simulink model "simulink_control"  (R2024a)
settings: Solver=ode5  StartTime=0.0  StopTime=inf  FixedStep=0.016  RelTol=1e-3
values from neighbouring files (symbols this model uses):
  hip = wb_robot_get_device('hip')    [inverted_pendulum_noncart.m]
  horizontal_motor = wb_robot_get_device('horizontal_motor')    [inverted_pendulum_noncart.m]
  horizontal_position_sensor = wb_robot_get_device('horizontal position sensor')    [inverted_pendulum_noncart.m]
  TIME_STEP = 16    [inverted_pendulum_noncart.m]
undefined symbols (not defined in the file or in its folder): a1, a2, a3, a4, accelerometer_sensor
libraries: slpidlib x2, eeGeneralControl x1, simulink_extras x1
settings Model: Creator=Harun  LastModifiedBy=Harun

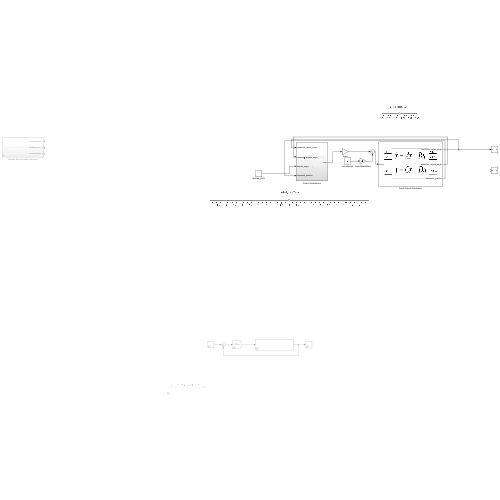
[thumbnail: Simulink's stored preview of the top-level diagram]
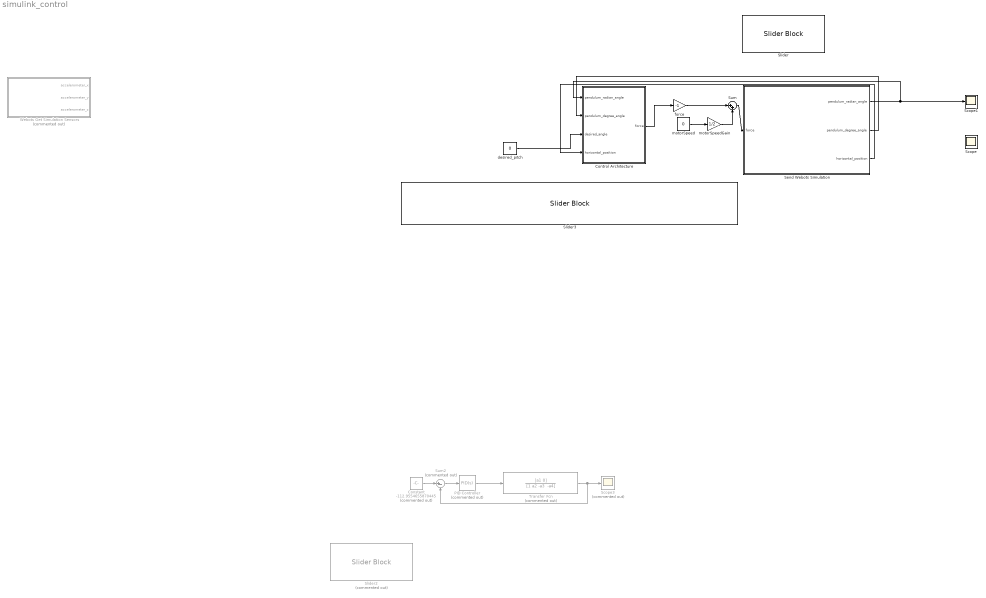
== system simulink_control ==
  Constant : Constant  Commented=on  Value=-112.9554655870445
  Control Architecture : Subsystem
  PID Controller : slpidlib/PID Controller  Commented=on  Controller=PID  Form=Parallel  TimeDomain=Continuous-time  UseExternalTs=off  SampleTime=-1  IntegratorMethod=Forward Euler  FilterMethod=Forward Euler  ControllerParametersSource=internal  P=117.155618821838  I=67.2944879318419  UseKiTs=off  D=44.7801205202101  UseExternalDerivativeSource=off  N=97.4887289682428  UseFilter=on  TunerSelectOption=Transfer Function Based (PID Tuner App)  InitialConditionSource=internal  InitialConditionForIntegrator=0  InitialConditionForFilter=0  DifferentiatorICPrevScaledInput=0  ExternalReset=none  TrackingMode=off  Kt=1  LimitOutput=off  SatLimitsSource=internal  UpperSaturationLimit=inf  LowerSaturationLimit=-inf  LinearizeAsGain=on  AntiWindupMode=none  Kb=1  LimitIntegrator=off  UpperIntegratorSaturationLimit=inf  LowerIntegratorSaturationLimit=-inf  POutMin=[]  POutMax=[]  IOutMin=[]  IOutMax=[]  DOutMin=[]  DOutMax=[]  NOutMin=[]  NOutMax=[]  SumOutMin=[]  SumOutMax=[]  SaturationOutMin=[]  SaturationOutMax=[]  PParamMin=[]  PParamMax=[]  IParamMin=[]  IParamMax=[]  DParamMin=[]  DParamMax=[]  NParamMin=[]  NParamMax=[]  KbParamMin=[]  KbParamMax=[]  KtParamMin=[]  KtParamMax=[]  KbOutMin=[]  KbOutMax=[]  KtOutMin=[]  KtOutMax=[]  IntegratorOutMin=[]  IntegratorOutMax=[]  FilterOutMin=[]  FilterOutMax=[]  SumI1OutMin=[]  SumI1OutMax=[]  SumI2OutMin=[]  SumI2OutMax=[]  SumI3OutMin=[]  SumI3OutMax=[]  SumI4OutMin=[]  SumI4OutMax=[]  SumDOutMin=[]  SumDOutMax=[]  DifferentiatorOutMin=[]  DifferentiatorOutMax=[]  FilterDiffOutCoefMin=[]  FilterDiffOutCoefMax=[]  ReciprocalOutMin=[]  ReciprocalOutMax=[]  SumDenOutMin=[]  SumDenOutMax=[]  SumNumOutMin=[]  SumNumOutMax=[]  DivideOutMin=[]  DivideOutMax=[]  UdiffTsProdOutMin=[]  UdiffTsProdOutMax=[]  NTsProdOutMin=[]  NTsProdOutMax=[]  UintegralTsProdOutMin=[]  UintegralTsProdOutMax=[]  UngainTsProdOutMin=[]  UngainTsProdOutMax=[]  ClampingZeroOutDataTypeStr=Inherit: Inherit via back propagation  ClampingZeroOutMin=[]  ClampingZeroOutMax=[]  FilterDenConstantOutDataTypeStr=Inherit: Inherit via back propagation  FilterDenConstantOutMin=[]  FilterDenConstantOutMax=[]  PCopyOutDataTypeStr=Inherit: Inherit via back propagation  PCopyOutMin=[]  PCopyOutMax=[]  NCopyOutDataTypeStr=Inherit: Inherit via back propagation  NCopyOutMin=[]  NCopyOutMax=[]  IntegratorContinuousStateAttributes=''  IntegratorStateMustResolveToSignalObject=off  IntegratorRTWStateStorageClass=Auto  FilterContinuousStateAttributes=''  FilterStateMustResolveToSignalObject=off  FilterRTWStateStorageClass=Auto  ParallelPVariant=InternalParameters  IdealPVariant=Disabled  IVariant=InternalParameters  DVariant=InternalParameters  IntegratorVariant=Continuous  SatVariant=Disabled  AWVariant=Passthrough  PCopyVariant=Disabled  TRVariant=Disabled  FdbkBlocksVariant=Forward  IdealPFdbkVariant=Disabled  SatFdbkVariant=Disabled  DerivativeFilterVariant=ContFilter  NVariant=InternalParameters  NCopyVariant=Disabled  FilterICVariant=InternalICsFilter  IntegratorICVariant=InternalICs  ExternalResetVariant=Disabled  TRSumVariant=Passthrough  SumFdbkVariant=Disabled  SumVariant=Sum_PID  TsampFilterVariant=InternalTs  TsampNgainVariant=Passthrough  TsampIntegralVariant=Passthrough  ExternalSaturationOutDataTypeStr=Inherit: Same as second input  DerivativeSourceVariant=ErrorSignal
  Scope : Scope
  Scope1 : Scope
  Scope3 : Scope  Commented=on
  Send Webots Simulation : Subsystem
      mask Display: image('./block_images/webots_plant_model.png');
  Slider : SliderBlock  ScaleMin=-9.99  ScaleMax=9.99
  Slider2 : SliderBlock  Commented=on  ScaleMin=-180  ScaleMax=180
  Slider3 : SliderBlock  ScaleMin=-5  ScaleMax=5
  Sum : Sum  Inputs=|++
  Sum2 : Sum  Commented=on  Inputs=|+-
  Transfer Fcn : TransferFcn  Commented=on  Numerator=[a1 0]  Denominator="[1 a2 -a3  -a4]"
  Webots Get Simulation Sensors : Subsystem  Commented=on
  desired_pitch : Constant  Value=0
  force : Gain  Gain=-1
  motorSpeed : Constant  Value=0
  motorSpeedGain : Gain  Gain=1/2
  wires:
  motorSpeed/1 -> motorSpeedGain/1
  Sum/1 -> Send Webots Simulation/1(force)
  Control Architecture/1(force) -> force/1
  motorSpeedGain/1 -> Sum/2
  Send Webots Simulation/1(pendulum_radian_angle) -> Scope1/1, Control Architecture/1(pendulum_radian_angle)
  force/1 -> Sum/1
  PID Controller/1 -> Transfer Fcn/1
  Sum2/1 -> PID Controller/1
  Constant/1 -> Sum2/1
  Transfer Fcn/1 -> Scope3/1, Sum2/2
  desired_pitch/1 -> Control Architecture/3(desired_angle)
  Send Webots Simulation/2(pendulum_degree_angle) -> Control Architecture/2(pendulum_degree_angle)
  Send Webots Simulation/3(horizontal_position) -> Control Architecture/4(horizontal_position)

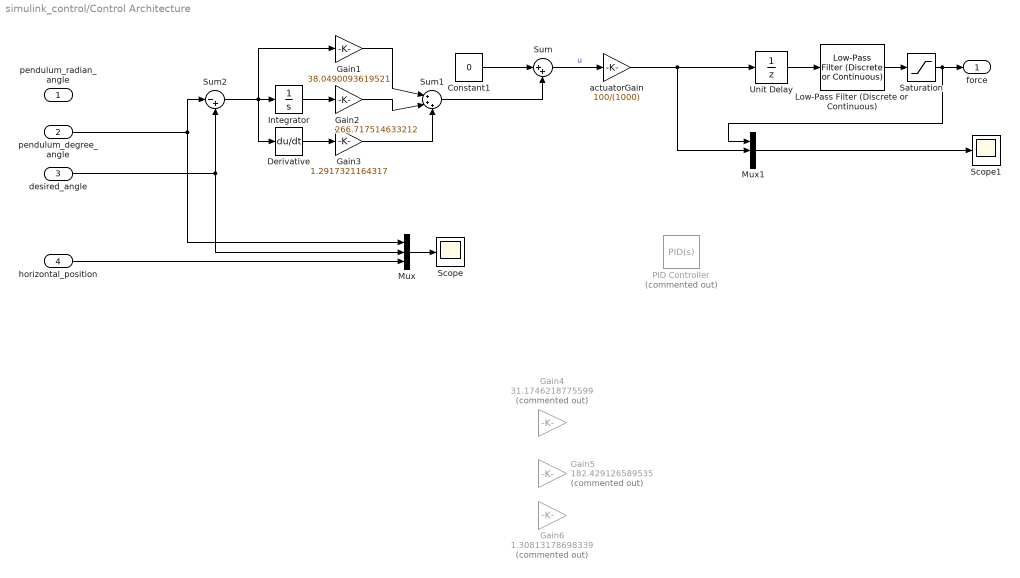
== system simulink_control/Control Architecture ==
  pendulum_radian_angle : Inport
  pendulum_degree_angle : Inport  Port=2
  desired_angle : Inport  Port=3
  horizontal_position : Inport  Port=4
  Constant1 : Constant  Value=0
  Derivative : Derivative  CoefficientInTFapproximation=0.016
  Gain1 : Gain  Gain=38.0490093619521
  Gain2 : Gain  Gain=266.717514633212
  Gain3 : Gain  Gain=1.2917321164317
  Gain4 : Gain  Commented=on  Gain=31.1746218775599
  Gain5 : Gain  Commented=on  Gain=182.429126589535
  Gain6 : Gain  Commented=on  Gain=1.30813178698339
  Integrator : Integrator  AbsoluteTolerance=0.016
  Low-Pass Filter (Discrete or Continuous) : eeGeneralControl/Low-Pass Filter (Discrete or Continuous)  K=1  T=0.016  B=inf  A=-inf  init_option=Inherited from block input  x0=0  Ts=-1
  Mux : Mux  Inputs=3
  Mux1 : Mux  Inputs=3
  PID Controller : slpidlib/PID Controller  Commented=on  Controller=PID  Form=Parallel  TimeDomain=Continuous-time  UseExternalTs=off  SampleTime=-1  IntegratorMethod=Forward Euler  FilterMethod=Forward Euler  ControllerParametersSource=internal  P=2.84315843974577  I=4.99760643504796  UseKiTs=off  D=0.397176332191921  UseExternalDerivativeSource=off  N=204.781529595043  UseFilter=on  TunerSelectOption=Transfer Function Based (PID Tuner App)  InitialConditionSource=internal  InitialConditionForIntegrator=0  InitialConditionForFilter=0  DifferentiatorICPrevScaledInput=0  ExternalReset=none  TrackingMode=off  Kt=1  LimitOutput=off  SatLimitsSource=internal  UpperSaturationLimit=inf  LowerSaturationLimit=-inf  LinearizeAsGain=on  AntiWindupMode=none  Kb=1  LimitIntegrator=off  UpperIntegratorSaturationLimit=inf  LowerIntegratorSaturationLimit=-inf  POutMin=[]  POutMax=[]  IOutMin=[]  IOutMax=[]  DOutMin=[]  DOutMax=[]  NOutMin=[]  NOutMax=[]  SumOutMin=[]  SumOutMax=[]  SaturationOutMin=[]  SaturationOutMax=[]  PParamMin=[]  PParamMax=[]  IParamMin=[]  IParamMax=[]  DParamMin=[]  DParamMax=[]  NParamMin=[]  NParamMax=[]  KbParamMin=[]  KbParamMax=[]  KtParamMin=[]  KtParamMax=[]  KbOutMin=[]  KbOutMax=[]  KtOutMin=[]  KtOutMax=[]  IntegratorOutMin=[]  IntegratorOutMax=[]  FilterOutMin=[]  FilterOutMax=[]  SumI1OutMin=[]  SumI1OutMax=[]  SumI2OutMin=[]  SumI2OutMax=[]  SumI3OutMin=[]  SumI3OutMax=[]  SumI4OutMin=[]  SumI4OutMax=[]  SumDOutMin=[]  SumDOutMax=[]  DifferentiatorOutMin=[]  DifferentiatorOutMax=[]  FilterDiffOutCoefMin=[]  FilterDiffOutCoefMax=[]  ReciprocalOutMin=[]  ReciprocalOutMax=[]  SumDenOutMin=[]  SumDenOutMax=[]  SumNumOutMin=[]  SumNumOutMax=[]  DivideOutMin=[]  DivideOutMax=[]  UdiffTsProdOutMin=[]  UdiffTsProdOutMax=[]  NTsProdOutMin=[]  NTsProdOutMax=[]  UintegralTsProdOutMin=[]  UintegralTsProdOutMax=[]  UngainTsProdOutMin=[]  UngainTsProdOutMax=[]  ClampingZeroOutDataTypeStr=Inherit: Inherit via back propagation  ClampingZeroOutMin=[]  ClampingZeroOutMax=[]  FilterDenConstantOutDataTypeStr=Inherit: Inherit via back propagation  FilterDenConstantOutMin=[]  FilterDenConstantOutMax=[]  PCopyOutDataTypeStr=Inherit: Inherit via back propagation  PCopyOutMin=[]  PCopyOutMax=[]  NCopyOutDataTypeStr=Inherit: Inherit via back propagation  NCopyOutMin=[]  NCopyOutMax=[]  IntegratorContinuousStateAttributes=''  IntegratorStateMustResolveToSignalObject=off  IntegratorRTWStateStorageClass=Auto  FilterContinuousStateAttributes=''  FilterStateMustResolveToSignalObject=off  FilterRTWStateStorageClass=Auto  ParallelPVariant=InternalParameters  IdealPVariant=Disabled  IVariant=InternalParameters  DVariant=InternalParameters  IntegratorVariant=Continuous  SatVariant=Disabled  AWVariant=Passthrough  PCopyVariant=Disabled  TRVariant=Disabled  FdbkBlocksVariant=Forward  IdealPFdbkVariant=Disabled  SatFdbkVariant=Disabled  DerivativeFilterVariant=ContFilter  NVariant=InternalParameters  NCopyVariant=Disabled  FilterICVariant=InternalICsFilter  IntegratorICVariant=InternalICs  ExternalResetVariant=Disabled  TRSumVariant=Passthrough  SumFdbkVariant=Disabled  SumVariant=Sum_PID  TsampFilterVariant=InternalTs  TsampNgainVariant=Passthrough  TsampIntegralVariant=Disabled_SignalSpec  ExternalSaturationOutDataTypeStr=Inherit: Same as second input  DerivativeSourceVariant=ErrorSignal
  Saturation : Saturate  UpperLimit=100  LowerLimit=-100
  Scope : Scope
  Scope1 : Scope
  Sum : Sum  Inputs=|++
  Sum1 : Sum  Inputs=|+++
  Sum2 : Sum  Inputs=|-+
  Unit Delay : UnitDelay  SampleTime=-1  HasFrameUpgradeWarning=on
  actuatorGain : Gain  Gain=100/(1000)
  force : Outport
  wires:
  pendulum_degree_angle/1 -> Sum2/1, Mux/1
  Constant1/1 -> Sum/1
  Sum/1 -> actuatorGain/1  "u"
  Unit Delay/1 -> Low-Pass Filter (Discrete or Continuous)/1
  horizontal_position/1 -> Mux/3
  Mux/1 -> Scope/1
  Sum2/1 -> Gain1/1, Derivative/1, Integrator/1
  Mux1/1 -> Scope1/1
  Gain1/1 -> Sum1/1
  Integrator/1 -> Gain2/1
  Gain2/1 -> Sum1/2
  Low-Pass Filter (Discrete or Continuous)/1 -> Saturation/1
  Saturation/1 -> Mux1/1, force/1
  actuatorGain/1 -> Mux1/2, Unit Delay/1
  Sum1/1 -> Sum/2
  Derivative/1 -> Gain3/1
  Gain3/1 -> Sum1/3
  ? -> Gain4/1
  ? -> Gain6/1
  ? -> Gain5/1
  desired_angle/1 -> Sum2/2, Mux/2

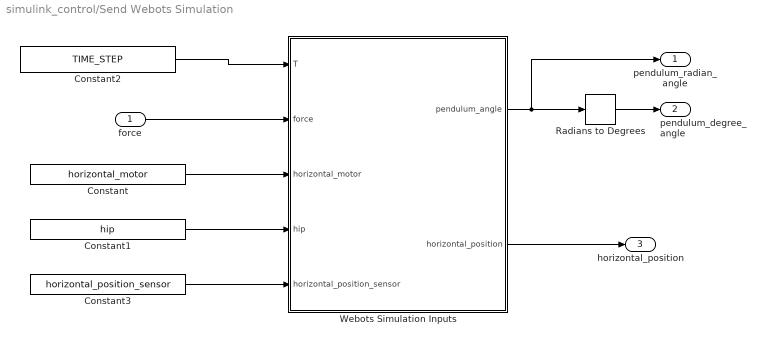
== system simulink_control/Send Webots Simulation ==
  force : Inport
  Constant : Constant  Value=horizontal_motor
  Constant1 : Constant  Value=hip
  Constant2 : Constant  Value=TIME_STEP
  Constant3 : Constant  Value=horizontal_position_sensor
  Radians to Degrees : simulink_extras/Transformations/Radians to Degrees
  Webots Simulation Inputs : MATLAB Function  TreatAsAtomicUnit=on
  pendulum_radian_angle : Outport
  pendulum_degree_angle : Outport  Port=2
  horizontal_position : Outport  Port=3
  wires:
  Constant2/1 -> Webots Simulation Inputs/1(T)
  Webots Simulation Inputs/1(pendulum_angle) -> Radians to Degrees/1, pendulum_radian_angle/1
  Radians to Degrees/1 -> pendulum_degree_angle/1
  Webots Simulation Inputs/2(horizontal_position) -> horizontal_position/1
  force/1 -> Webots Simulation Inputs/2(force)
  Constant/1 -> Webots Simulation Inputs/3(horizontal_motor)
  Constant1/1 -> Webots Simulation Inputs/4(hip)
  Constant3/1 -> Webots Simulation Inputs/5(horizontal_position_sensor)

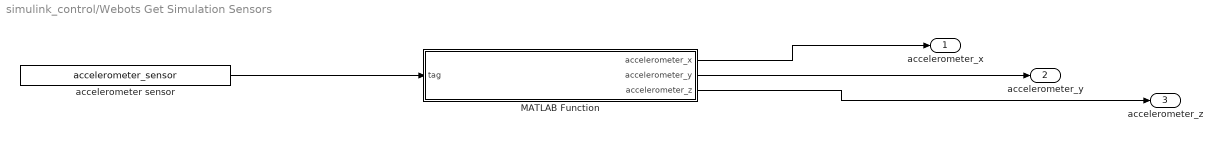
== system simulink_control/Webots Get Simulation Sensors ==
  MATLAB Function : MATLAB Function  TreatAsAtomicUnit=on
  accelerometer sensor : Constant  Value=accelerometer_sensor
  accelerometer_x : Outport
  accelerometer_y : Outport  Port=2
  accelerometer_z : Outport  Port=3
  wires:
  accelerometer sensor/1 -> MATLAB Function/1(tag)
  MATLAB Function/1(accelerometer_x) -> accelerometer_x/1
  MATLAB Function/3(accelerometer_z) -> accelerometer_z/1
  MATLAB Function/2(accelerometer_y) -> accelerometer_y/1

== matlab function simulink_control/Webots Get Simulation Sensors/MATLAB Function ==
  data: tag input; accelerometer_x output; accelerometer_y output; accelerometer_z output
function [accelerometer_x,accelerometer_y,accelerometer_z] = accelerometer_sensor_get(tag)

period = wb_accelerometer_get_sampling_period(tag)
values = wb_accelerometer_get_values(tag);
accelerometer_x = values(1);
accelerometer_y = values(2);
accelerometer_z = values(3);

== matlab function simulink_control/Send Webots Simulation/Webots Simulation Inputs ==
  data: T input; force input; horizontal_motor input; hip input; horizontal_position_sensor input; pendulum_angle output; horizontal_position output
function [pendulum_angle,horizontal_position]  =   simulation(T,force,horizontal_motor,hip,horizontal_position_sensor)



wb_robot_step(T)

wb_motor_set_force(horizontal_motor,force);

pendulum_angle=0.0;
horizontal_position=0.0;
horizontal_position1 = wb_position_sensor_get_value(horizontal_position_sensor);
horizontal_position=horizontal_position1;
hip_value = wb_position_sensor_get_value(hip);
pendulum_angle = hip_value;

end
